simulink model "matlab3"  (R2018b)
settings: Solver=VariableStepAuto  StartTime=0.0  StopTime=100  RelTol=1e-3
libraries: simulink x1
settings Model: Creator=stud  LastModifiedBy=groinder
settings DebuggingCC: LibraryContextMissingDiagnostic=none
settings SFSimCC: SimUseLocalCustomCode=off
settings RTWCC: RTWUseLocalCustomCode=off

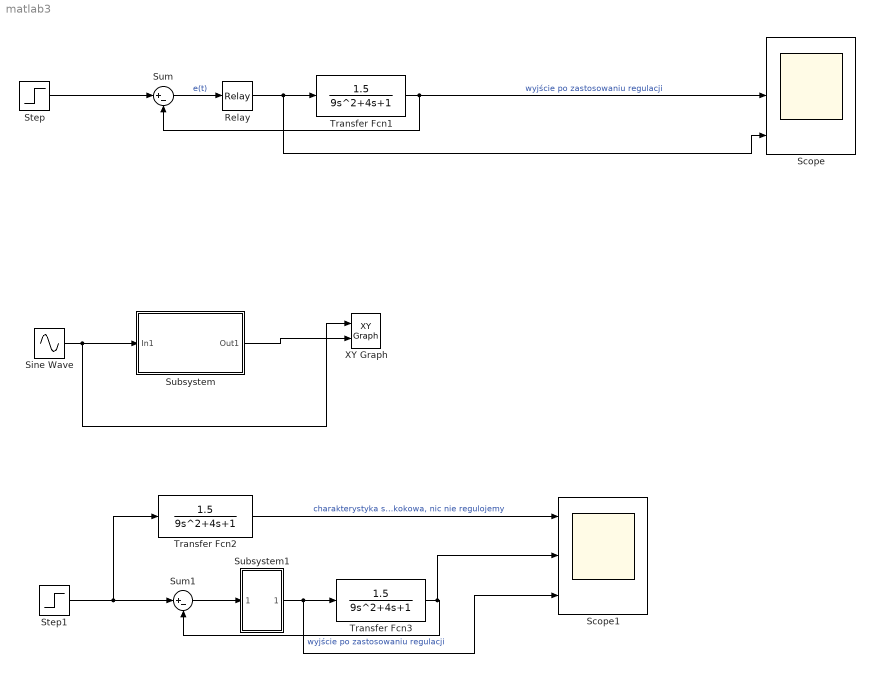
== system matlab3 ==
  Relay : Relay  OnSwitchValue=0  OffSwitchValue=0
  Scope : Scope  NumInputPorts=3
  Scope1 : Scope  NumInputPorts=3
  Sine Wave : Sin  SampleTime=0
  Step : Step  SampleTime=0
  Step1 : Step  SampleTime=0
  Subsystem : Subsystem
  Subsystem1 : Subsystem
  Sum : Sum  Inputs=|+-
  Sum1 : Sum  Inputs=|+-
  Transfer Fcn1 : TransferFcn  Numerator=[1.5]  Denominator=[9 4 1]
  Transfer Fcn2 : TransferFcn  Numerator=[1.5]  Denominator=[9 4 1]
  Transfer Fcn3 : TransferFcn  Numerator=[1.5]  Denominator=[9 4 1]
  XY Graph : simulink/Sinks/XY Graph  xmin=-1  xmax=1  ymin=-1  ymax=1  st=-1
  wires:
  Step/1 -> Sum/1
  Sum/1 -> Relay/1  "e(t)"
  Relay/1 -> Scope/3, Transfer Fcn1/1
  Transfer Fcn1/1 -> Scope/2, Sum/2  "wyjście po zastosowaniu regulacji"
  Sine Wave/1 -> Subsystem/1(In1), XY Graph/1
  Subsystem/1(Out1) -> XY Graph/2
  Transfer Fcn3/1 -> Scope1/2, Sum1/2  "wyjście po zastosowaniu regulacji"
  Step1/1 -> Sum1/1, Transfer Fcn2/1
  Sum1/1 -> Subsystem1/1(In1)
  Subsystem1/1(Out1) -> Scope1/3, Transfer Fcn3/1
  Transfer Fcn2/1 -> Scope1/1  "charakterystyka skokowa, nic nie regulojemy"

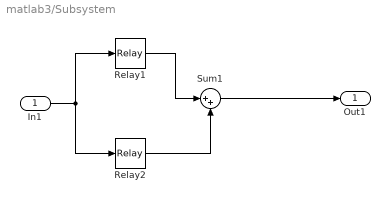
== system matlab3/Subsystem ==
  In1 : Inport
  Relay1 : Relay  OnSwitchValue=0.5  OffSwitchValue=0.2
  Relay2 : Relay  OnSwitchValue=-0.2  OffSwitchValue=-0.5  OnOutputValue=0  OffOutputValue=-1
  Sum1 : Sum  Inputs=|++
  Out1 : Outport
  wires:
  Relay2/1 -> Sum1/2
  Sum1/1 -> Out1/1
  In1/1 -> Relay2/1, Relay1/1
  Relay1/1 -> Sum1/1

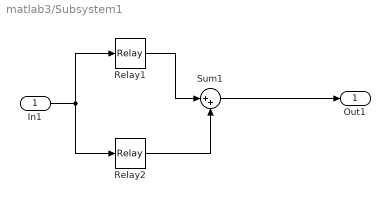
== system matlab3/Subsystem1 ==
  In1 : Inport
  Relay1 : Relay  OnSwitchValue=0.5  OffSwitchValue=0.2
  Relay2 : Relay  OnSwitchValue=-0.2  OffSwitchValue=-0.5  OnOutputValue=0  OffOutputValue=-1
  Sum1 : Sum  Inputs=|++
  Out1 : Outport
  wires:
  Relay2/1 -> Sum1/2
  Sum1/1 -> Out1/1
  In1/1 -> Relay2/1, Relay1/1
  Relay1/1 -> Sum1/1
